simulink model "Quaternions_Method_merge_gio_giusto"  (R2021b)
settings: Solver=FixedStepAuto  StartTime=0.0  StopTime=Time  FixedStep=1  RelTol=1e-13  AbsTol=1e-8
values from neighbouring files (symbols this model uses):
  a = 8.6251e+06    (= 8625100)    [Main.m]
  c = 299792*10^3    (= 299792000)    [Main.m]
  e = 0.1195    [Main.m]
  G = 6.67259 * 1e-11    (= 6.67259e-11)    [Main.m]
  H_0 = sqrt((g_1_0)^2 + (g_1_1)^2 + (h_1_1)^2)    [Main.m]
  i = 0.3815    [Main.m]
  MB = [2000; 0.3; 1; 0.12].*1e-2    [Main.m]
  mr = 1.2 * 0.0001    (= 0.00012)    [Main.m]
  muP = G*Mt    (= 398527110340000)    [Main.m]
  omega_0 = [om_x, om_y, om_z]    [Main.m]
  p_acc = deg2rad(5)    [Main.m]
  RD = 0.1*ones(1,10)    [Main.m]
  RS_MB = 0.5    [Main.m]
  RS_SP = 0.1    [Main.m]
  SP = [2000; 0.3; 1; 0.12].*1e-2    [Main.m]
  theta0 = 0    [Main.m]
  w_E = (2*pi)/(24*3600)    (= 7.27220521664e-05)    [Main.m]
undefined symbols (not defined in the file or in its folder): A_BN_0, A_rw, A_rw_star, H, magnitude, rho_d_MB, rho_d_SP, rho_s_MB, rho_s_SP, sig_b, sig_n, T, t_sample
libraries: matrix_library x23, vrlib x9, simulink_extras x2, simulink x2
(part 1 of 8)
settings Model: SimulationMode=accelerator  Creator=dario  LastModifiedBy=adity
settings SolverCC: ZeroCrossControl=DisableAll  ZeroCrossAlgorithm=Adaptive  AlgebraicLoopSolver=TrustRegion
settings DebuggingCC: IgnoredZcDiagnostic=none

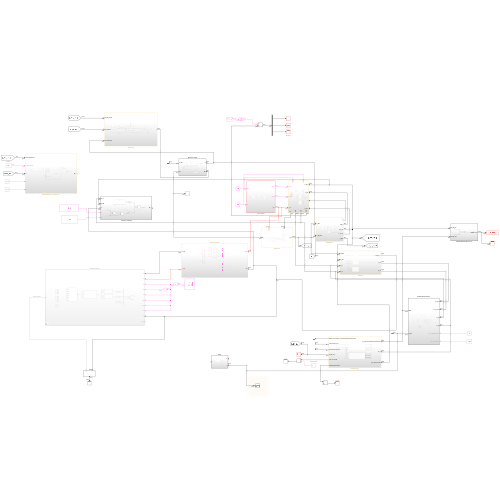
[thumbnail: Simulink's stored preview of the top-level diagram]
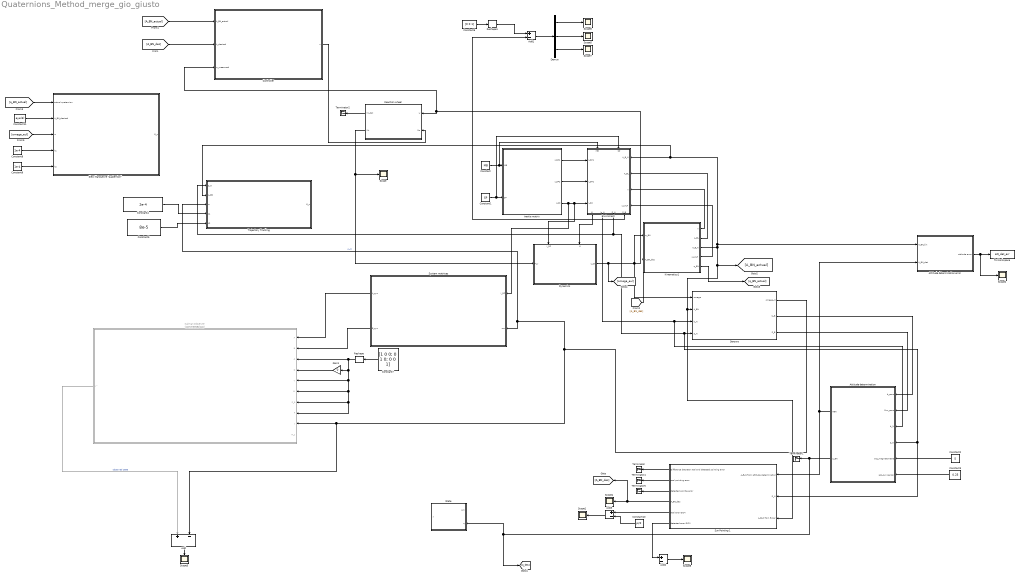
== system Quaternions_Method_merge_gio_giusto ==
  Add{,1..3} (4 alike) : Sum  Inputs=+-
  Attitude determination : Subsystem
  Attitude determination error : Subsystem
  Constant : Constant  Value=MB
  Constant1 : Constant  Value=SP
  Constant10 : Constant  Value=pi/2
  Constant11 : Constant  Value=eye(3)
  Constant2 : Constant  Value=5
  Constant3 : Constant  Value=0.25
  Constant4 : Constant  Value=2e-4
  Constant5 : Constant  Value=8e-5
  Constant6 : Constant  Value=[0 0 1]  VectorParams1D=off
  Constant7 : Constant  Value=[1 0 0; 0 1 0; 0 0 1]  VectorParams1D=off
  Constant8 : Constant  Value=1e-4
  Constant9 : Constant  Value=1e-4
  Controller : Subsystem
  Demux : Demux  Outputs=3
  Dynamics : Subsystem
      settings: PortSchema="{\"entries\":[{\"content\":{\"sides\":[{\"content\":{\"connectorIds\":[\"In1\"]},\"type\":\"ConnectorPlacement.EquallySpacedRectSide\",\"uuid\":\"0fb0fd28-732a-45b7-951f-4b0b2306202c\"},{\"content\":{\"connectorIds\":[\"Out1\"],\"side\":\"RIGHT\"},\"type\":\"ConnectorPlacement.EquallySpacedRectSide\",\"uuid\":\"160a6d95-5e8b-4088-9ac4-372e2ef53b1e\"},{\"content\":{\"connectorIds\":[\"In2\",\"In3\"],\"side\":\"TOP\"},\"type\":\"ConnectorPlacement.EquallySpacedRectSide\",\"uuid\":\"bc0d773d-9b3c-40c2-804a-fc9efd6e220c\"}]},\"type\":\"ConnectorPlacement.EquallySpacedConnector\",\"uuid\":\"1f85a25c-c8d4-4d9d-9994-483d99135538\"}],\"packageUris\":[\"http://schema.mathworks.com/mf0/Connector/R2020b\"],\"version\":\"1.0\"}"
  Enviroment : Subsystem
      settings: PortSchema="{\"entries\":[{\"content\":{\"sides\":[{\"content\":{\"connectorIds\":[\"In1\",\"In2\"]},\"type\":\"ConnectorPlacement.EquallySpacedRectSide\",\"uuid\":\"77a65197-c5ef-4c05-af97-bd670bb59a1b\"},{\"content\":{\"connectorIds\":[\"Out1\",\"Out2\",\"Out3\",\"Out4\"],\"side\":\"RIGHT\"},\"type\":\"ConnectorPlacement.EquallySpacedRectSide\",\"uuid\":\"f4905732-994b-44e8-915f-1f1165b6d340\"},{\"content\":{\"connectorIds\":[\"In3\",\"In4\",\"In5\"],\"side\":\"TOP\"},\"type\":\"ConnectorPlacement.EquallySpacedRectSide\",\"uuid\":\"dbb628bc-072b-4daa-a580-a056bf799753\"},{\"content\":{\"connectorIds\":[\"In6\",\"In7\",\"In8\",\"In9\"],\"side\":\"BOTTOM\"},\"type\":\"ConnectorPlacement.EquallySpacedRectSide\",\"uuid\":\"e6af6235-b92e-4098-9bbc-91b77f168ead\"}]},\"type\":\"ConnectorPlacement.EquallySpacedConnector\",\"uuid\":\"a4645f0d-8f51-4ba7-9ec5-d423e83ccc17\"}],\"packageUris\":[\"http://schema.mathworks.com/mf0/Connector/R2020b\"],\"version\":\"1.0\"}"
  Gain1 : Gain  Gain=0
  Inertia matrix : Subsystem
  Kalman Observer : Subsystem  Commented=on
  Kinematics1 : Subsystem
  Reaction wheel : Subsystem
  Reshape : Reshape  OutputDimensionality=Customize  OutputDimensions=[3,3]
  Reshape1 : Reshape  OutputDimensionality=Column vector (2-D)
  Scope{,1..8} (9 alike) : Scope
  Sensors : Subsystem
  "Slew Manouevre \"quaternion\"" : Subsystem
  State : Subsystem
  Sun Pointing 1 : Subsystem
  System matrices : Subsystem
  Terminator{,1..2,4..5} (5 alike) : Terminator
  To Workspace : ToWorkspace  VariableName=att_det_err  SaveFormat=Timeseries  SampleTime=-1
  Trajectory Tracking : Subsystem
  wires:
  Enviroment/1(M) -> Dynamics/3(M)
  Kinematics1/2(A_BL) -> Enviroment/7(A_BL)
  Kinematics1/1(n) -> Enviroment/8(n)
  Constant/1 -> Inertia matrix/1(MB), Enviroment/1(MB)
  Constant1/1 -> Inertia matrix/2(SP), Enviroment/2(SP)
  Inertia matrix/1(r_SP1) -> Enviroment/3(r_SP1)
  Inertia matrix/2(r_SP2) -> Enviroment/4(r_SP2)
  Dynamics/1(ω_B) -> [omega_eul], Controller/3(w_measured), Reaction wheel/1(w), Kinematics1/1(ω_BN), Sensors/1(omega)
  Inertia matrix/3(I_SC) -> System matrices/1(I_SC), Enviroment/5(I_SC), Dynamics/2(I_SC)
  Sensors/1(omega_m) -> Add/2, Kalman Observer/9(x), Trajectory Tracking/3(" ω"), System matrices/2(om)  "w_m"
  Enviroment/2(b_N) -> Attitude determination/3(b_N), Sensors/3(b_N)
  Enviroment/3(S_N) -> Sun Pointing 1/2(S_N), Attitude determination/4(S_N), Sensors/4(S_N), Trajectory Tracking/1(S_N)
  Constant3/1 -> Attitude determination/6(acc_sun sensor)
  Attitude determination/1(ABN) -> Attitude determination error/2(A_BN_det), Sun Pointing 1/1(A_B_N from attitude determination)
  Sensors/2(b_B) -> Attitude determination/1(b_sens)
  Attitude determination/2(q_BN) -> State/2(q), [q_des], Terminator1/1
  Constant2/1 -> Attitude determination/5(acc_magnetometre)
  Sensors/3(S_B) -> Attitude determination/2(Sun_sens)
  Sun Pointing 1/3(detected pointig error) -> Terminator5/1
  Sun Pointing 1/2(real pointing error) -> Terminator4/1
  Sun Pointing 1/1(Difference between real and detected pointing error) -> Terminator/1
  Kinematics1/4(r_LVLH) -> Enviroment/9(r_LVLH)
  Attitude determination error/1(attitude error) -> Scope2/1, To Workspace/1
  System matrices/1(A_sys) -> Kalman Observer/1(A)
  System matrices/2(B_sys) -> Kalman Observer/2(B)
  Constant7/1 -> Reshape/1
  Gain1/1 -> Kalman Observer/4(D)
  Kalman Observer/1(x^) -> Add/1  "observed state"
  Add/1 -> Scope3/1
  Reshape/1 -> Kalman Observer/3(C), Gain1/1, Kalman Observer/5(V), Kalman Observer/6(W), Kalman Observer/7(P_0), Kalman Observer/8(F)
  Constant4/1 -> Trajectory Tracking/4(k1)
  Constant5/1 -> Trajectory Tracking/5(k2)
  Reaction wheel/2(Mr) -> Dynamics/1(M_r), Scope/1
  Reaction wheel/1(hr_dot) -> Terminator2/1
  Sun Pointing 1/4(A_BN_des) -> [A_BN_des], Scope4/1
  [A_BN_des] -> Controller/2(A_desired)
  [A_BN_actual] -> Controller/1(A_BN_actual)
  Controller/1(u) -> Reaction wheel/2(Mc)
  Kinematics1/3(A_B_N) -> Sun Pointing 1/3(A_B_N from Euler), Sensors/2(A_BN), [A_BN_actual], Trajectory Tracking/2(A_BN), Enviroment/6(A_B_N), Attitude determination error/1(A_BN_kin)
  Constant6/1 -> Reshape1/1
  Enviroment/4(S_B) -> Add1/2
  Reshape1/1 -> Add1/1
  Add1/1 -> Demux/1
  Demux/2 -> Scope5/1
  Demux/1 -> Scope6/1
  Demux/3 -> Scope7/1
  [A_BN_des] -> Kinematics1/2(A_BN_des)
  Sun Pointing 1/6(detected error DCM) -> Add2/1
  Add2/1 -> Scope8/1
  Kinematics1/5(q_BN) -> [q_BN_actual]
  [q_BN_actual] -> "Slew Manouevre \"quaternion\""/1(actual quaternion)
  Constant11/1 -> "Slew Manouevre \"quaternion\""/2(A_BN_desired)
  [omega_eul] -> "Slew Manouevre \"quaternion\""/3(ω)
  Constant9/1 -> "Slew Manouevre \"quaternion\""/5(k2)
  Constant8/1 -> "Slew Manouevre \"quaternion\""/4(k1)
  Sun Pointing 1/5(real error DCM) -> Add3/1
  Add3/1 -> Scope1/1
  Constant10/1 -> Add3/2

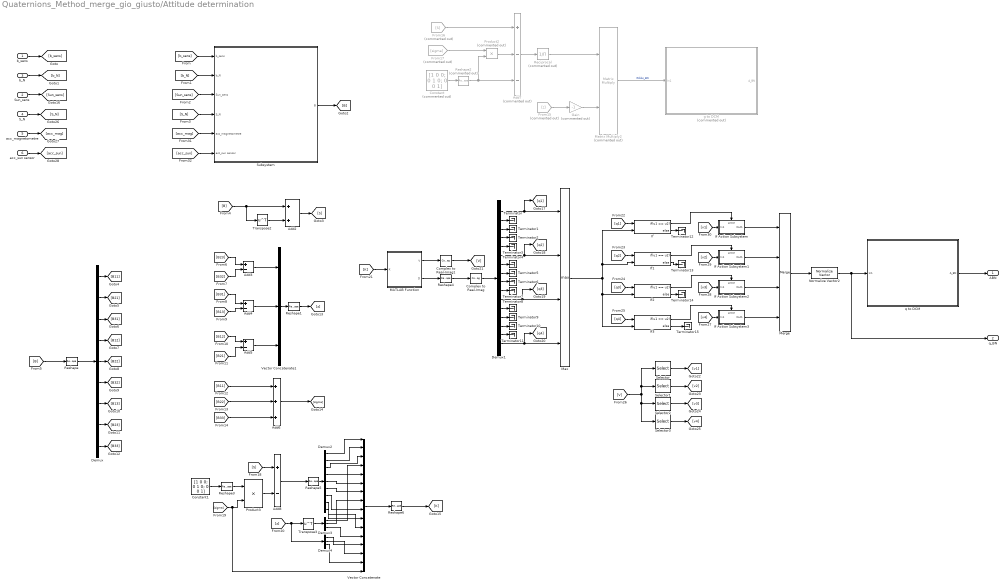
== system Quaternions_Method_merge_gio_giusto/Attitude determination ==
  b_sens : Inport
  Sun_sens : Inport  Port=2
  b_N : Inport  Port=3
  S_N : Inport  Port=4
  acc_magnetometre : Inport  Port=5
  acc_sun sensor : Inport  Port=6
  Add2 : Sum
  Add{3..5,8} (4 alike) : Sum  Inputs=+-
  Add6 : Sum  Inputs=+++
  Add7 : Sum  Commented=on  Inputs=+--
  Complex to Real-Imag : ComplexToRealImag  Output=Real
  Complex to Real-Imag1 : ComplexToRealImag  Output=Real
  Constant : Constant  Commented=on  Value=[1 0 0; 0 1 0; 0 0 1]  VectorParams1D=off
  Constant1 : Constant  Value=[1 0 0; 0 1 0; 0 0 1]  VectorParams1D=off
  Demux : Demux  Outputs=9
  Demux1 : Demux  Outputs=16
  Demux2 : Demux  Outputs=9
  Demux3 : Demux  Outputs=3
  Demux4 : Demux  Outputs=3
  From15 : From  Commented=on  GotoTag=z
  From16 : From  Commented=on  GotoTag=S
  From17 : From  Commented=on  GotoTag=sigma
  Gain : Gain  Commented=on  Gain=-1
  If{,1..3} (4 alike) : If  NumInputs=2  IfExpression=u1 == u2
  If Action Subsystem : Subsystem  TreatAsAtomicUnit=on
  If Action Subsystem1 : Subsystem  TreatAsAtomicUnit=on
  If Action Subsystem2 : Subsystem  TreatAsAtomicUnit=on
  If Action Subsystem3 : Subsystem  TreatAsAtomicUnit=on
  MATLAB Function : MATLAB Function  TreatAsAtomicUnit=on
  Matrix Multiply2 : Product  Commented=on  Multiplication=Matrix(*)
  Max : MinMax  Function=max  Inputs=4
  Merge : Merge  Inputs=4
  Normalize Vector2 : vrlib/Utilities/Normalize Vector  maxzero=0
  Product2 : Product  Commented=on
  Product3 : Product
  Reciprocal : Product  Commented=on  Inputs=/
  Reshape{,1,4..5} (4 alike) : Reshape  OutputDimensionality=Column vector (2-D)
  Reshape2 : Reshape  Commented=on  OutputDimensionality=Customize  OutputDimensions=[3,3]
  Reshape3 : Reshape  OutputDimensionality=Customize  OutputDimensions=[3,3]
  Reshape6 : Reshape  OutputDimensionality=Customize  OutputDimensions=[4,4]
  Selector : Selector  NumberOfDimensions=2  InputPortWidth=3  IndexOptions=Index vector (dialog),Index vector (dialog)  Indices=[1 2 3 4],1  OutputSizes=1,1
  Selector1 : Selector  NumberOfDimensions=2  InputPortWidth=3  IndexOptions=Index vector (dialog),Index vector (dialog)  Indices=[1 2 3 4],2  OutputSizes=1,1
  Selector2 : Selector  NumberOfDimensions=2  InputPortWidth=3  IndexOptions=Index vector (dialog),Index vector (dialog)  Indices=[1 2 3 4],3  OutputSizes=1,1
  Selector3 : Selector  NumberOfDimensions=2  InputPortWidth=3  IndexOptions=Index vector (dialog),Index vector (dialog)  Indices=[1 2 3 4],4  OutputSizes=1,1
  Subsystem : Subsystem
  Terminator{,1..15} (16 alike) : Terminator
  Transpose2 : Math  Operator=transpose  SaturateOnIntegerOverflow=on
  Transpose3 : Math  Operator=transpose  SaturateOnIntegerOverflow=on
  Vector Concatenate : Concatenate  NumInputs=16
  Vector Concatenate1 : Concatenate  NumInputs=3
  g to DCM : Subsystem  Commented=on
  q to DCM : Subsystem
  ABN : Outport
  q_BN : Outport  Port=2
  wires:
  [B] -> Transpose2/1, Add2/1
  Transpose2/1 -> Add2/2
  Add2/1 -> [S]
  [B] -> Reshape/1
  Reshape/1 -> Demux/1
  Demux/1 -> [B11]
  Demux/2 -> [B21]
  Demux/3 -> [B31]
  Demux/4 -> [B12]
  Demux/5 -> [B22]
  Demux/6 -> [B32]
  Demux/7 -> [B13]
  Demux/8 -> [B23]
  Demux/9 -> [B33]
  [B23] -> Add3/1
  [B32] -> Add3/2
  [B31] -> Add4/1
  [B13] -> Add4/2
  [B12] -> Add5/1
  [B21] -> Add5/2
  Add3/1 -> Vector Concatenate1/1
  Add4/1 -> Vector Concatenate1/2
  Add5/1 -> Vector Concatenate1/3
  Vector Concatenate1/1 -> Reshape1/1
  Reshape1/1 -> [z]
  [B11] -> Add6/1
  [B22] -> Add6/2
  [B33] -> Add6/3
  Add6/1 -> [sigma]
  From15/1 -> Gain/1
  Constant/1 -> Reshape2/1
  From17/1 -> Product2/1
  Reshape2/1 -> Add7/3, Product2/2
  From16/1 -> Add7/1
  Product2/1 -> Add7/2
  Add7/1 -> Reciprocal/1
  Reciprocal/1 -> Matrix Multiply2/1
  Gain/1 -> Matrix Multiply2/2
  Matrix Multiply2/1 -> g to DCM/1(In1)  "Gibbs_BN"
  Constant1/1 -> Reshape3/1
  Reshape3/1 -> Product3/1
  [sigma] -> Vector Concatenate/16, Product3/2
  Product3/1 -> Add8/2
  [S] -> Add8/1
  Add8/1 -> Reshape5/1
  MATLAB Function/2(D) -> Reshape4/1
  Demux1/2 -> Terminator/1
  Demux1/3 -> Terminator1/1
  Demux1/4 -> Terminator2/1
  Demux1/5 -> Terminator3/1
  Demux1/6 -> [q2], Max/2
  Demux1/7 -> Terminator4/1
  Demux1/8 -> Terminator5/1
  Demux1/9 -> Terminator6/1
  Demux1/10 -> Terminator7/1
  Demux1/11 -> [q3], Max/3
  Demux1/16 -> [q4], Max/4
  Demux1/12 -> Terminator8/1
  Demux1/13 -> Terminator9/1
  Demux1/14 -> Terminator10/1
  Demux1/15 -> Terminator11/1
  Reshape4/1 -> Complex to Real-Imag/1
  Max/1 -> If3/2, If2/2, If1/2, If/2
  Demux1/1 -> [q1], Max/1
  [q1] -> If/1
  [q2] -> If1/1
  [q4] -> If3/1
  [q3] -> If2/1
  MATLAB Function/1(V) -> Complex to Real-Imag1/1
  Selector1/1 -> [v2]
  Selector3/1 -> [v4]
  Selector2/1 -> [v3]
  Selector/1 -> [v1]
  [V] -> Selector/1, Selector1/1, Selector3/1, Selector2/1
  If/1 -> If Action Subsystem/Action
  If/2 -> Terminator12/1
  If1/2 -> Terminator13/1
  If2/2 -> Terminator14/1
  If3/2 -> Terminator15/1
  If Action Subsystem/1(Out1) -> Merge/1
  If1/1 -> If Action Subsystem1/Action
  If2/1 -> If Action Subsystem2/Action
  If3/1 -> If Action Subsystem3/Action
  If Action Subsystem3/1(Out1) -> Merge/4
  If Action Subsystem2/1(Out1) -> Merge/3
  If Action Subsystem1/1(Out1) -> Merge/2
  [v4] -> If Action Subsystem3/1(In1)
  [v1] -> If Action Subsystem/1(In1)
  [v2] -> If Action Subsystem1/1(In1)
  [v3] -> If Action Subsystem2/1(In1)
  q to DCM/1(A_BN) -> ABN/1
  Merge/1 -> Normalize Vector2/1
  Reshape5/1 -> Demux2/1
  Demux2/1 -> Vector Concatenate/1
  Demux2/2 -> Vector Concatenate/2
  Demux2/3 -> Vector Concatenate/3
  [z] -> Demux4/1, Transpose3/1
  Transpose3/1 -> Demux3/1
  Demux3/1 -> Vector Concatenate/4
  Demux2/4 -> Vector Concatenate/5
  Demux2/5 -> Vector Concatenate/6
  Demux2/6 -> Vector Concatenate/7
  Demux3/2 -> Vector Concatenate/8
  Demux2/7 -> Vector Concatenate/9
  Demux2/8 -> Vector Concatenate/10
  Demux2/9 -> Vector Concatenate/11
  Demux3/3 -> Vector Concatenate/12
  Demux4/2 -> Vector Concatenate/14
  Demux4/1 -> Vector Concatenate/13
  Demux4/3 -> Vector Concatenate/15
  Vector Concatenate/1 -> Reshape6/1
  Reshape6/1 -> [K]
  Complex to Real-Imag/1 -> Demux1/1
  Normalize Vector2/1 -> q_BN/1, q to DCM/1(In1)
  Complex to Real-Imag1/1 -> [V]
  [K] -> MATLAB Function/1(K)
  Subsystem/1(B) -> [B]
  b_sens/1 -> [b_sens]
  b_N/1 -> [b_N]
  Sun_sens/1 -> [Sun_sens]
  S_N/1 -> [S_N]
  acc_magnetometre/1 -> [acc_mag]
  acc_sun sensor/1 -> [acc_sun]
  [b_sens] -> Subsystem/1(b_sens)
  [b_N] -> Subsystem/2(b_N)
  [Sun_sens] -> Subsystem/3(Sun_sens)
  [S_N] -> Subsystem/4(S_N)
  [acc_mag] -> Subsystem/5(acc_magnetometre)
  [acc_sun] -> Subsystem/6(acc_sun sensor)

== system Quaternions_Method_merge_gio_giusto/Attitude determination error ==
  A_BN_kin : Inport
  A_BN_det : Inport  Port=2
  Add : Sum  Inputs=+-
  attitude error : Outport
  wires:
  Add/1 -> attitude error/1
  A_BN_kin/1 -> Add/2
  A_BN_det/1 -> Add/1

== system Quaternions_Method_merge_gio_giusto/Controller ==
  A_BN_actual : Inport
  A_desired : Inport  Port=2
  w_measured : Inport  Port=3
  -k1 : Gain  Gain=-3*10^-5
  -k2 : Gain  Gain=-3*10^-5
  Gain : Gain  Gain=-1
  Matrix Multiply : Product  Multiplication=Matrix(*)
  Mux : Mux  Inputs=3
  Reshape : Reshape  OutputDimensionality=Customize  OutputDimensions=[3,1]
  Scope{,1..3} (4 alike) : Scope
  Selector : Selector  NumberOfDimensions=2  InputPortWidth=3  IndexOptions=Index vector (dialog),Index vector (dialog)  Indices=2,1  OutputSizes=1,1
  Selector1 : Selector  NumberOfDimensions=2  InputPortWidth=3  IndexOptions=Index vector (dialog),Index vector (dialog)  Indices=3,1  OutputSizes=1,1
  Selector2 : Selector  NumberOfDimensions=2  InputPortWidth=3  IndexOptions=Index vector (dialog),Index vector (dialog)  Indices=3,2  OutputSizes=1,1
  Sum : Sum  Inputs=|+|-|
  Sum1 : Sum  Inputs=|+|+|
  Transpose1 : Math  Operator=transpose  SaturateOnIntegerOverflow=on
  u : Outport
  wires:
  A_desired/1 -> Matrix Multiply/2
  A_BN_actual/1 -> Matrix Multiply/1
  Matrix Multiply/1 -> Scope/1, Sum/2, Transpose1/1
  Transpose1/1 -> Sum/1
  Sum/1 -> Selector2/1, Selector/1, Selector1/1
  Mux/1 -> Reshape/1
  Selector1/1 -> Gain/1
  Selector/1 -> Scope3/1, Mux/1
  Selector2/1 -> Mux/3
  -k2/1 -> Sum1/1
  Sum1/1 -> Scope2/1, u/1
  w_measured/1 -> Scope1/1, -k1/1
  -k1/1 -> Sum1/2
  Reshape/1 -> -k2/1
  Gain/1 -> Mux/2

== system Quaternions_Method_merge_gio_giusto/Dynamics ==
  M_r : Inport
  I_SC : Inport  Port=2
  M : Inport  Port=3
  Add : Sum
  Constant7 : Constant  Value=omega_0
  Cross Product : vrlib/Utilities/Cross Product
  Demux : Demux  Outputs=3
  Gain5 : Gain  Gain=-1
  Integrator4 : Integrator  InitialConditionSource=external  InitialCondition=omega_0
  Product6 : Product  Multiplication=Matrix(*)
  Product7 : Product  Multiplication=Matrix(*)
  Reciprocal : Product  Inputs=/  Multiplication=Matrix(*)
  Scope : Scope  NumInputPorts=3
  Sum2 : Sum
  Terminator : Terminator
  ω_B : Outport
  wires:
  Sum2/1 -> Product7/2
  Product6/1 -> Cross Product/2
  Product7/1 -> Terminator/1, Integrator4/1
  Cross Product/1 -> Gain5/1
  Gain5/1 -> Sum2/1
  Integrator4/1 -> Demux/1, Cross Product/1, Product6/2, ω_B/1
  I_SC/1 -> [I_SC]
  [I_SC] -> Product6/1
  [I_SC] -> Reciprocal/1
  Reciprocal/1 -> Product7/1
  Constant7/1 -> [w_0]
  [w_0] -> Integrator4/2
  M/1 -> Add/1
  Demux/2 -> Scope/2  "om_y"
  Demux/1 -> Scope/1  "om_x"
  Demux/3 -> Scope/3  "om_z"
  Add/1 -> Sum2/2
  M_r/1 -> Add/2

== system Quaternions_Method_merge_gio_giusto/Enviroment ==
  MB : Inport
  SP : Inport  Port=2
  r_SP1 : Inport  Port=3
  r_SP2 : Inport  Port=4
  I_SC : Inport  Port=5
  A_B_N : Inport  Port=6
  A_BL : Inport  Port=7
  n : Inport  Port=8
  r_LVLH : Inport  Port=9
  Constant : Constant  Value=6371.2*1e3
  Gravity gradient torque : Subsystem
  "Magnetic torque " : Subsystem
  Scope : Scope
  Scope1 : Scope
  Scope2 : Scope
  Solar Radiation Perturbation : Subsystem  Commented=on
  Solar Radiation Perturbation1 : Subsystem
  Sum : Sum  Inputs=+|+|+
  M : Outport
  b_N : Outport  Port=2
  S_N : Outport  Port=3
  S_B : Outport  Port=4
  wires:
  A_B_N/1 -> Solar Radiation Perturbation1/1(A_B_N), "Magnetic torque "/2(A_B_N)
  MB/1 -> Solar Radiation Perturbation1/2(MB)
  SP/1 -> Solar Radiation Perturbation1/3(SP)
  r_SP1/1 -> Solar Radiation Perturbation1/4(r_SP1)
  r_SP2/1 -> Solar Radiation Perturbation1/5(r_SP2)
  Sum/1 -> M/1
  Solar Radiation Perturbation1/1(M_SRP) -> Scope/1, Sum/2
  "Magnetic torque "/1(M) -> Scope2/1, Sum/3
  Constant/1 -> "Magnetic torque "/1(R)
  Gravity gradient torque/1(M_GG) -> Scope1/1, Sum/1
  I_SC/1 -> Gravity gradient torque/1(I)
  n/1 -> Gravity gradient torque/3(n)
  A_BL/1 -> Gravity gradient torque/2(A_BL)
  "Magnetic torque "/2(b_N) -> [b_N]
  [b_N] -> b_N/1
  Solar Radiation Perturbation1/2(S_N) -> [S_N]
  [S_N] -> S_N/1
  r_LVLH/1 -> "Magnetic torque "/3(r_LVLH)
  Solar Radiation Perturbation1/3(S_B) -> S_B/1

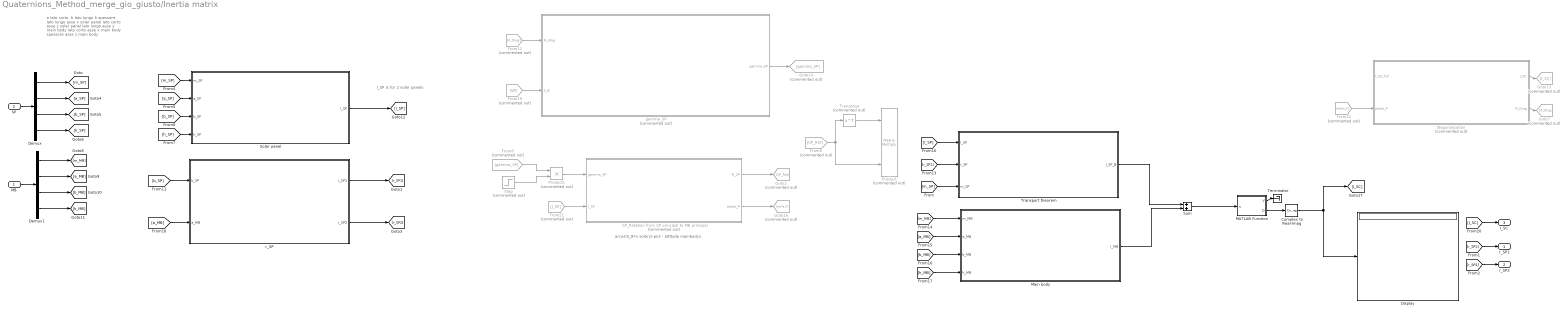
== system Quaternions_Method_merge_gio_giusto/Inertia matrix ==
  note: I_SP is for 2 solar panels
  note: arcos(S_B*n solary)-pi/2 - attitude mainbodyx
  note: a lato corto, b lato lungo h spessore
      | lato lungo asse x solar panel
      | lato corto asse z solar panel
      | lato lungo asse y main body
      | lato corto asse x main body
      | spessore asse z main body
  MB : Inport
  SP : Inport  Port=2
  Complex to Real-Imag : ComplexToRealImag  Output=Real
  Demux : Demux
  Demux1 : Demux
  Diagonalization : Subsystem  Commented=on
  Display : Display
  From12 : From  Commented=on  GotoTag=R_Diag
  From19 : From  Commented=on  GotoTag=SB
  From21 : From  Commented=on  GotoTag=I_SP
  From22 : From  Commented=on  GotoTag=alpha_P
  From8 : From  Commented=on  GotoTag=gamma_SP
  From9 : From  Commented=on  GotoTag=SP_Rot
  Goto13 : Goto  Commented=on  GotoTag=I_SC
  Goto14 : Goto  Commented=on  GotoTag=gamma_SP
  Goto16 : Goto  Commented=on  GotoTag=alpha_P
  Goto2 : Goto  Commented=on  GotoTag=SP_Rot
  Goto7 : Goto  Commented=on  GotoTag=R_Diag
  MATLAB Function : MATLAB Function  TreatAsAtomicUnit=on
  Main body : Subsystem
  Product : Product  Commented=on  Inputs=3  Multiplication=Matrix(*)
  Product1 : Product  Commented=on
  SP_Rotation from SP principal to MB principal : Subsystem  Commented=on
  Solar panel : Subsystem
  Step : Step  Commented=on  Time=1e-3  SampleTime=0
  Sum : Sum
  Terminator : Terminator
  Transport theorem : Subsystem
  Transpose : Math  Commented=on  Operator=transpose  SaturateOnIntegerOverflow=on
  gamma_SP : Subsystem  Commented=on
  r_SP : Subsystem
  r_SP1 : Outport
  r_SP2 : Outport  Port=2
  I_SC : Outport  Port=3
  wires:
  MB/1 -> Demux1/1
  Demux/1 -> [m_SP]
  SP_Rotation from SP principal to MB principal/1(R_SP) -> Goto2/1
  Transpose/1 -> Product/1
  Transport theorem/1(I_SP_B) -> Sum/1
  [r_SP1] -> Transport theorem/2(r_SP)
  Main body/1(I_MB) -> Sum/2
  [m_SP] -> Transport theorem/3(m_SP)
  r_SP/1(r_SP1) -> [r_SP1]
  [r_SP1] -> r_SP1/1
  [r_SP2] -> r_SP2/1
  r_SP/2(r_SP2) -> [r_SP2]
  Demux/2 -> [a_SP]
  Demux/3 -> [b_SP]
  Demux/4 -> [h_SP]
  [a_SP] -> Solar panel/2(a_SP)
  [b_SP] -> Solar panel/3(b_SP)
  [m_SP] -> Solar panel/1(m_SP)
  [h_SP] -> Solar panel/4(h_SP)
  From9/1 -> Transpose/1, Product/3
  [b_SP] -> r_SP/1(b_SP)
  Demux1/4 -> [h_MB]
  Demux1/3 -> [b_MB]
  Demux1/2 -> [a_MB]
  Demux1/1 -> [m_MB]
  [m_MB] -> Main body/1(m_MB)
  [a_MB] -> Main body/2(a_MB)
  [b_MB] -> Main body/3(b_MB)
  [h_MB] -> Main body/4(h_MB)
  [a_MB] -> r_SP/2(a_MB)
  Solar panel/1(I_SP) -> [I_SP]
  Product1/1 -> SP_Rotation from SP principal to MB principal/1(gamma_SP)
  From8/1 -> Product1/1
  Step/1 -> Product1/2
  SP/1 -> Demux/1
  Diagonalization/2(R_Diag) -> Goto7/1
  From12/1 -> gamma_SP/1(R_diag)
  From19/1 -> gamma_SP/2(S_B)
  Diagonalization/1(I_SC) -> Goto13/1
  [I_SC] -> I_SC/1
  gamma_SP/1(gamma_SP) -> Goto14/1
  From21/1 -> SP_Rotation from SP principal to MB principal/2(I_SP)
  SP_Rotation from SP principal to MB principal/2(alpha_P) -> Goto16/1
  From22/1 -> Diagonalization/2(alpha_P)
  [I_SP] -> Transport theorem/1(I_SP)
  Sum/1 -> MATLAB Function/1(u)
  MATLAB Function/1(V) -> Terminator/1
  MATLAB Function/2(D) -> Complex to Real-Imag/1
  Complex to Real-Imag/1 -> [I_SC], Display/1

== system Quaternions_Method_merge_gio_giusto/Kalman Observer ==
  A : Inport
  B : Inport  Port=2
  C : Inport  Port=3
  D : Inport  Port=4
  V : Inport  Port=5
  W : Inport  Port=6
  P_0 : Inport  Port=7
  F : Inport  Port=8
  x : Inport  Port=9
  M_c : Inport  Port=10
  A^ : Subsystem
  Add : Sum  Inputs=+++
  B^ : Subsystem
  Integrator : Integrator  InitialConditionSource=external
  L : Subsystem
  Matrix Multiply : Product  Multiplication=Matrix(*)
  Matrix Multiply1 : Product  Multiplication=Matrix(*)
  Matrix Multiply2 : Product  Multiplication=Matrix(*)
  Riccati : Subsystem
  x^ : Outport
  wires:
  A/1 -> [A]
  V/1 -> [V]
  B/1 -> [B]
  W/1 -> [W]
  F/1 -> [F]
  [A] -> Riccati/1(A)
  [F] -> Riccati/3(F)
  [W] -> Riccati/4(W)
  [V] -> Riccati/5(V)
  [B] -> B^/1(B)
  [L] -> B^/2(L)
  C/1 -> [C]
  [C] -> Riccati/2(C)
  L/1(L) -> [L]
  [P] -> L/1(P)
  Riccati/1(P) -> [P]
  [C] -> L/2(C)
  [V] -> L/3(V)
  [A] -> A^/1(A)
  [L] -> A^/2(L)
  x/1 -> [x]
  A^/1(A^) -> Matrix Multiply/1
  [x_obs] -> Matrix Multiply/2
  B^/1(B^) -> Matrix Multiply1/1
  M_c/1 -> [M_c]
  [M_c] -> Matrix Multiply1/2
  Matrix Multiply1/1 -> Add/1
  Matrix Multiply/1 -> Add/2
  Add/1 -> Integrator/1
  Integrator/1 -> [x_obs], x^/1
  [L] -> Matrix Multiply2/1
  [x] -> Matrix Multiply2/2
  [x] -> Integrator/2
  P_0/1 -> [P_0]
  [P_0] -> Riccati/6(P_0)
  D/1 -> [D]
  [D] -> B^/3(D)
  [C] -> A^/3(C)
  Matrix Multiply2/1 -> Add/3

== system Quaternions_Method_merge_gio_giusto/Kinematics1 ==
  ω_BN : Inport
  A_BN_des : Inport  Port=2
  Creazione Matrice A_BN : Subsystem
  Creazione quaternione : Subsystem
  MatrixMultiply : Product  Multiplication=Matrix(*)
  Orbit Propagation : Subsystem
  Relative_Attitude : Subsystem
  n : Outport
  A_BL : Outport  Port=2
  A_B_N : Outport  Port=3
  r_LVLH : Outport  Port=4
  q_BN : Outport  Port=5
  wires:
  Creazione Matrice A_BN/1(A_BN) -> A_B_N/1, Relative_Attitude/1(A_BN), Orbit Propagation/1(A_BN)
  ω_BN/1 -> Creazione quaternione/1(ω_BN)
  Creazione quaternione/1(q_normalizzato) -> q_BN/1, Creazione Matrice A_BN/1(q_normalizzato)
  Relative_Attitude/1(A_BL) -> A_BL/1
  Orbit Propagation/2(n) -> n/1
  Orbit Propagation/1(theta) -> Relative_Attitude/2(theta)
  Relative_Attitude/2(A_L/N) -> [A_LN]
  Orbit Propagation/3(r_N) -> MatrixMultiply/2
  [A_LN] -> MatrixMultiply/1
  MatrixMultiply/1 -> r_LVLH/1
  A_BN_des/1 -> Creazione quaternione/2(A_BN_des)

== system Quaternions_Method_merge_gio_giusto/Reaction wheel ==
  w : Inport
  Mc : Inport  Port=2
  A : Constant  Value=A_rw
  A_star : Constant  Value=A_rw_star
  Constant : Constant  Value=[0 0 0 0]
  Cross Product : matrix_library/Cross Product
      settings: SourceProductBaseCode=SL
  Gain : Gain  Gain=-1
  Integrator : Integrator  InitialConditionSource=external
  Matrix Multiply : Product  Multiplication=Matrix(*)
  Matrix Multiply1 : Product  Multiplication=Matrix(*)
  Matrix Multiply2 : Product  Multiplication=Matrix(*)
  Reshape : Reshape  OutputDimensionality=Column vector (2-D)
  Reshape1 : Reshape  OutputDimensionality=Column vector (2-D)
  Sum : Sum  Inputs=|++
  hr_dot : Outport
  Mr : Outport  Port=2
  wires:
  Integrator/1 -> Matrix Multiply/2
  A/1 -> [A_rw], Matrix Multiply/1
  w/1 -> Cross Product/1
  Matrix Multiply/1 -> Cross Product/2
  Cross Product/1 -> Sum/1
  Mc/1 -> Reshape1/1
  Sum/1 -> Matrix Multiply1/2
  A_star/1 -> Gain/1
  Gain/1 -> Matrix Multiply1/1
  Matrix Multiply1/1 -> Integrator/1, Matrix Multiply2/2, hr_dot/1
  Constant/1 -> Reshape/1
  Reshape/1 -> Integrator/2
  Reshape1/1 -> Sum/2
  Matrix Multiply2/1 -> Mr/1
  [A_rw] -> Matrix Multiply2/1

== system Quaternions_Method_merge_gio_giusto/Sensors ==
  omega : Inport
  A_BN : Inport  Port=2
  b_N : Inport  Port=3
  S_N : Inport  Port=4
  Gyroscopes : Subsystem
  Magnetometer1 : Subsystem
  Sun sensor : Subsystem
  omega_m : Outport
  b_B : Outport  Port=2
  S_B : Outport  Port=3
  wires:
  omega/1 -> Gyroscopes/1(omega)
  Gyroscopes/1(omega_m) -> omega_m/1
  b_N/1 -> Magnetometer1/2(b_N)
  Magnetometer1/1(b_B) -> b_B/1
  Sun sensor/1(S_B) -> S_B/1
  A_BN/1 -> Sun sensor/2(A_BN), Magnetometer1/1(A_BN)
  S_N/1 -> Sun sensor/1(S_N)

== system Quaternions_Method_merge_gio_giusto/Slew Manouevre "quaternion" ==
  actual quaternion : Inport
  A_BN_desired : Inport  Port=2
  ω : Inport  Port=3
  k1 : Inport  Port=4
  k2 : Inport  Port=5
  A_BN to quaternion : Subsystem
  Creation of Q_euler1 : Subsystem
  Demux : Demux
  Gain : Gain  Gain=-1
  Gain1 : Gain  Gain=-2
  Mux : Mux  Inputs=3
  Product : Product  Multiplication=Matrix(*)
  Product1 : Product
  Product2 : Product  Inputs=3
  Reshape : Reshape  OutputDimensionality=Column vector (2-D)
  Scope : Scope
  Sum : Sum  Inputs=|+|+|
  M_c : Outport
  wires:
  actual quaternion/1 -> Product/2
  Creation of Q_euler1/1(Q_desired) -> Product/1
  A_BN_desired/1 -> A_BN to quaternion/1(" A_BN_Desiderd")
  A_BN to quaternion/1(q_desiderd) -> Creation of Q_euler1/1(q_desired)
  k1/1 -> Gain/1
  Gain/1 -> Product1/1
  ω/1 -> Product1/2
  k2/1 -> Product2/1
  [q_error] -> Product2/3
  Product1/1 -> Sum/1
  Product2/1 -> Sum/2
  Sum/1 -> M_c/1
  Product/1 -> Scope/1, Demux/1
  Demux/1 -> [qe1]
  Demux/4 -> [qe4]
  Demux/3 -> [qe3]
  Demux/2 -> [qe2]
  [qe1] -> Mux/1
  [qe2] -> Mux/2
  [qe3] -> Mux/3
  Mux/1 -> Reshape/1
  Reshape/1 -> [q_error]
  [qe4] -> Gain1/1
  Gain1/1 -> Product2/2

== system Quaternions_Method_merge_gio_giusto/State ==
  om : Inport
  q : Inport  Port=2
  Reshape : Reshape  OutputDimensionality=Column vector (2-D)
  Vector Concatenate : Concatenate
  q to g : Subsystem
  x : Outport
  wires:
  q/1 -> q to g/1(q)
  om/1 -> Vector Concatenate/2
  q to g/1(g) -> Vector Concatenate/1
  Vector Concatenate/1 -> Reshape/1
  Reshape/1 -> x/1

== system Quaternions_Method_merge_gio_giusto/Sun Pointing 1 ==
  A_B_N from attitude determination : Inport
  S_N : Inport  Port=2
  A_B_N from Euler : Inport  Port=3
  Pointing error with DCM : Subsystem
  Pointing error with quaternions : Subsystem
  Difference between real and detected pointing error : Outport
  real pointing error : Outport  Port=2
  detected pointig error : Outport  Port=3
  A_BN_des : Outport  Port=4
  real error DCM : Outport  Port=5
  detected error DCM : Outport  Port=6
  wires:
  A_B_N from attitude determination/1 -> Pointing error with quaternions/1(A_B_N from attitude determination), Pointing error with DCM/3(A_B_N from Euler)
  S_N/1 -> Pointing error with quaternions/2(S_N), Pointing error with DCM/2(S_N)
  A_B_N from Euler/1 -> Pointing error with quaternions/3(A_B_N from Euler), Pointing error with DCM/1(A_B_N from attitude determination)
  Pointing error with DCM/1(Difference between real and detected pointing error) -> Difference between real and detected pointing error/1
  Pointing error with quaternions/2(detected pointing error) -> detected pointig error/1
  Pointing error with quaternions/1(real pointing error) -> real pointing error/1
  Pointing error with quaternions/3(q_euler) -> ?
  Pointing error with quaternions/4(q_desired) -> ?
  Pointing error with quaternions/5(A_BN_des) -> A_BN_des/1
  Pointing error with DCM/2(real error DCM) -> real error DCM/1
  Pointing error with DCM/3(Detected error DCM) -> detected error DCM/1

== system Quaternions_Method_merge_gio_giusto/System matrices ==
  I_SC : Inport
  om : Inport  Port=2
  Add : Sum  Inputs=+-
  Add1 : Sum  Inputs=+-
  Demux : Demux  Outputs=9
  Demux1 : Demux  Outputs=3
  Ground : Ground
  Ground1 : Ground
  Product{,1..3} (4 alike) : Product
  Reciprocal{,1..4} (5 alike) : Product  Inputs=/
  Reshape : Reshape
  Reshape1 : Reshape  OutputDimensionality=Customize  OutputDimensions=[3,3]
  Reshape2 : Reshape  OutputDimensionality=Customize  OutputDimensions=[3,3]
  Terminator{,1..7} (8 alike) : Terminator
  Vector Concatenate : Concatenate  NumInputs=9
  Vector Concatenate1 : Concatenate  NumInputs=9
  A_sys : Outport
  B_sys : Outport  Port=2
  wires:
  I_SC/1 -> Reshape/1
  Reshape/1 -> Demux/1
  Demux/1 -> [I_x]
  Demux/9 -> [I_z]
  Demux/5 -> [I_y]
  Demux/2 -> Terminator/1
  Demux/4 -> Terminator2/1
  Demux/3 -> Terminator1/1
  Demux/6 -> Terminator3/1
  Demux/7 -> Terminator4/1
  Demux/8 -> Terminator5/1
  [I_x] -> Reciprocal/1
  [I_y] -> Reciprocal1/1
  [I_z] -> Reciprocal2/1
  Reciprocal2/1 -> Vector Concatenate1/9
  Reciprocal1/1 -> Vector Concatenate1/5
  Reciprocal/1 -> Vector Concatenate1/1
  Vector Concatenate1/1 -> Reshape1/1
  Reshape1/1 -> B_sys/1
  om/1 -> Demux1/1
  Demux1/2 -> Terminator7/1
  Demux1/3 -> [om_z]
  Reshape2/1 -> A_sys/1
  Vector Concatenate/1 -> Reshape2/1
  Ground/1 -> Vector Concatenate/9, Vector Concatenate/8, Vector Concatenate/7, Vector Concatenate/6, Vector Concatenate/5, Vector Concatenate/3, Vector Concatenate/1
  [I_z] -> Add/1
  [I_x] -> Add/2
  [I_y] -> Reciprocal3/1
  Reciprocal3/1 -> Product/2
  Add/1 -> Product/1
  Add1/1 -> Product1/1
  Reciprocal4/1 -> Product1/2
  [I_z] -> Add1/2
  [I_y] -> Add1/1
  [I_x] -> Reciprocal4/1
  [A_21] -> Vector Concatenate/2
  [A_12] -> Vector Concatenate/4
  Demux1/1 -> Terminator6/1
  Product2/1 -> [A_21]
  Product/1 -> Product2/1
  [om_z] -> Product2/2
  [om_z] -> Product3/2
  Product1/1 -> Product3/1
  Product3/1 -> [A_12]
  Ground1/1 -> Vector Concatenate1/8, Vector Concatenate1/7, Vector Concatenate1/6, Vector Concatenate1/4, Vector Concatenate1/3, Vector Concatenate1/2

== system Quaternions_Method_merge_gio_giusto/Trajectory Tracking ==
  S_N : Inport
  A_BN : Inport  Port=2
  " ω" : Inport  Port=3
  k1 : Inport  Port=4
  k2 : Inport  Port=5
  Cross Product : matrix_library/Cross Product
      settings: SourceProductBaseCode=SL
  Gain : Gain  Gain=-1
  Gain1 : Gain  Gain=-1
  Matrix Multiply : Product  Multiplication=Matrix(*)
  Product : Product
  Product1 : Product
  Sum : Sum  Inputs=|+|+|
  M_c : Outport
  wires:
  S_N/1 -> Cross Product/2, Matrix Multiply/2
  A_BN/1 -> Matrix Multiply/1
  k1/1 -> Gain/1
  k2/1 -> Gain1/1
  Matrix Multiply/1 -> Cross Product/1
  Cross Product/1 -> Product/2
  Gain1/1 -> Product/1
  Gain/1 -> Product1/1
  " ω"/1 -> Product1/2
  Product1/1 -> Sum/1
  Product/1 -> Sum/2
  Sum/1 -> M_c/1

== system Quaternions_Method_merge_gio_giusto/Attitude determination/If Action Subsystem ==
  In1 : Inport
  Action Port : ActionPort  ActionPortLabel=if(u1 == u2)
  Out1 : Outport
  wires:
  In1/1 -> Out1/1

== system Quaternions_Method_merge_gio_giusto/Attitude determination/If Action Subsystem1 ==
  In1 : Inport
  Action Port : ActionPort  ActionPortLabel=if(u1 == u2)
  Out1 : Outport
  wires:
  In1/1 -> Out1/1

== system Quaternions_Method_merge_gio_giusto/Attitude determination/If Action Subsystem2 ==
  In1 : Inport
  Action Port : ActionPort  ActionPortLabel=if(u1 == u2)
  Out1 : Outport
  wires:
  In1/1 -> Out1/1

== system Quaternions_Method_merge_gio_giusto/Attitude determination/If Action Subsystem3 ==
  In1 : Inport
  Action Port : ActionPort  ActionPortLabel=if(u1 == u2)
  Out1 : Outport
  wires:
  In1/1 -> Out1/1

== system Quaternions_Method_merge_gio_giusto/Attitude determination/Subsystem ==
  b_sens : Inport
  b_N : Inport  Port=2
  Sun_sens : Inport  Port=3
  S_N : Inport  Port=4
  acc_magnetometre : Inport  Port=5
  acc_sun sensor : Inport  Port=6
  Add : Sum
  Add1 : Sum
  Divide : Product  Inputs=*/
  Divide1 : Product  Inputs=*/
  Matrix Multiply : Product  Multiplication=Matrix(*)
  Matrix Multiply1 : Product  Multiplication=Matrix(*)
  Normalize Vector : vrlib/Utilities/Normalize Vector  maxzero=0
  Normalize Vector1 : vrlib/Utilities/Normalize Vector  maxzero=0
  Product : Product
  Product1 : Product
  Transpose : Math  Operator=transpose  SaturateOnIntegerOverflow=on
  Transpose1 : Math  Operator=transpose  SaturateOnIntegerOverflow=on
  B : Outport
  wires:
  Transpose/1 -> Matrix Multiply1/2
  b_N/1 -> Normalize Vector1/1
  S_N/1 -> Transpose1/1
  Divide1/1 -> Product1/2
  Normalize Vector/1 -> Matrix Multiply1/1
  Add/1 -> B/1
  Divide/1 -> Product/2
  Product/1 -> Add/1
  b_sens/1 -> Normalize Vector/1
  Add1/1 -> Divide/2, Divide1/2
  [alpha2] -> Divide1/1
  [alpha1] -> Divide/1
  [alpha1] -> Add1/1
  Transpose1/1 -> Matrix Multiply/2
  acc_sun sensor/1 -> [alpha2]
  Matrix Multiply/1 -> Product1/1
  Matrix Multiply1/1 -> Product/1
  [alpha2] -> Add1/2
  acc_magnetometre/1 -> [alpha1]
  Normalize Vector1/1 -> Transpose/1
  Product1/1 -> Add/2
  Sun_sens/1 -> Matrix Multiply/1

== system Quaternions_Method_merge_gio_giusto/Attitude determination/g to DCM ==
  In1 : Inport
  A_BN : Outport
  wires:
  In1/1 -> A_BN/1

== system Quaternions_Method_merge_gio_giusto/Attitude determination/q to DCM ==
  In1 : Inport
  Add : Sum  Inputs=+-
  Add1 : Sum  Inputs=++-
  Constant : Constant  Value=[1 0 0; 0 1 0; 0 0 1]  VectorParams1D=off
  Demux : Demux
  Gain : Gain  Gain=2
  Gain1 : Gain  Gain=2
  Matrix Multiply : Product  Multiplication=Matrix(*)
  Matrix Multiply2 : Product  Multiplication=Matrix(*)
  Mux : Mux  Inputs=3
  Product : Product
  Product1 : Product
  Reshape : Reshape  OutputDimensionality=Column vector (2-D)
  Reshape1 : Reshape  OutputDimensionality=Customize  OutputDimensions=[3,3]
  Square : Math  Operator=square  SaturateOnIntegerOverflow=on
  Transpose : Math  Operator=transpose  SaturateOnIntegerOverflow=on
  Transpose1 : Math  Operator=transpose  SaturateOnIntegerOverflow=on
  q_cross : Subsystem
  A_BN : Outport
  wires:
  In1/1 -> Demux/1
  Demux/4 -> [q4]
  Demux/1 -> [q1]
  Demux/2 -> [q2]
  Demux/3 -> [q3]
  [q4] -> Square/1
  [q2] -> Mux/2
  [q3] -> Mux/3
  [q1] -> Mux/1
  Mux/1 -> Reshape/1
  Reshape/1 -> [q_vect]
  [q_vect] -> Matrix Multiply/2, Transpose/1
  Transpose/1 -> Matrix Multiply/1
  Matrix Multiply/1 -> Add/2
  Square/1 -> Add/1
  Constant/1 -> Reshape1/1
  Reshape1/1 -> Product1/2
  Product1/1 -> Add1/1
  Matrix Multiply2/1 -> Gain/1
  Gain/1 -> Add1/2
  Transpose1/1 -> Matrix Multiply2/2
  [q_vect] -> Transpose1/1, Matrix Multiply2/1
  Gain1/1 -> Add1/3
  Product/1 -> Gain1/1
  [q4] -> Product/2
  q_cross/1(q_cross) -> Product/1
  Add1/1 -> A_BN/1
  [q_vect] -> q_cross/1(q_vect)
  Add/1 -> Product1/1

== system Quaternions_Method_merge_gio_giusto/Enviroment/Gravity gradient torque ==
  I : Inport
  A_BL : Inport  Port=2
  n : Inport  Port=3
  Constant : Constant  Value=3
  Constant1 : Constant  Value=[1 0 0]
  Demux : Demux  Outputs=9
  Demux1 : Demux  Outputs=3
  Matrix Multiply : Product  Multiplication=Matrix(*)
  Mux : Mux  Inputs=3
  Product{,1..9} (10 alike) : Product
  Reshape : Reshape  OutputDimensionality=Column vector (2-D)
  Reshape1 : Reshape  OutputDimensionality=Column vector (2-D)
  Reshape2 : Reshape  OutputDimensionality=Column vector (2-D)
  Square : Math  Operator=square  SaturateOnIntegerOverflow=on
  Sum : Sum  Inputs=+-
  Sum1 : Sum  Inputs=+-
  Sum2 : Sum  Inputs=+-
  Terminator{,1..5} (6 alike) : Terminator
  M_GG : Outport
  wires:
  Demux/4 -> Terminator2/1
  n/1 -> Square/1
  Demux1/1 -> Product5/2, Product7/2
  Demux/2 -> Terminator/1
  Product6/1 -> Product9/1
  Sum/1 -> Product1/1
  Product1/1 -> Product6/1
  Demux/7 -> Terminator4/1
  Demux1/3 -> Product6/2, Product8/2
  Demux/1 -> Sum1/1
  Product5/1 -> Product8/1
  Demux/3 -> Terminator1/1
  I/1 -> Reshape1/1
  Matrix Multiply/1 -> Demux1/1
  Demux/9 -> Sum2/2, Sum1/2, Sum/1
  Constant1/1 -> Reshape/1
  Sum1/1 -> Product2/1
  Sum2/1 -> Product3/1
  Product7/1 -> Mux/3
  Mux/1 -> Reshape2/1
  Demux/5 -> Sum/2, Sum2/1
  Demux/8 -> Terminator5/1
  A_BL/1 -> Matrix Multiply/1
  Product4/1 -> Product7/1
  Product8/1 -> Mux/2
  Demux/6 -> Terminator3/1
  Demux1/2 -> Product4/2, Product9/2
  Product2/1 -> Product5/1
  Product9/1 -> Mux/1
  Product3/1 -> Product4/1
  Reshape/1 -> Matrix Multiply/2
  Reshape1/1 -> Demux/1
  Reshape2/1 -> M_GG/1
  Square/1 -> Product/1
  Product/1 -> Product2/2, Product1/2, Product3/2
  Constant/1 -> Product/2

== system Quaternions_Method_merge_gio_giusto/Enviroment/Magnetic torque  ==
  R : Inport
  A_B_N : Inport  Port=2
  r_LVLH : Inport  Port=3
  Creation of parasitic torque : Subsystem
  Cross Product : matrix_library/Cross Product
      settings: SourceProductBaseCode=SL
  Magnetic field in body frame : Subsystem
  M : Outport
  b_N : Outport  Port=2
  wires:
  R/1 -> Magnetic field in body frame/2(R)
  A_B_N/1 -> Magnetic field in body frame/1(A_B_N)
  Magnetic field in body frame/1(b_B) -> Cross Product/2
  Cross Product/1 -> M/1
  Creation of parasitic torque/1(m) -> Cross Product/1
  Magnetic field in body frame/2(b_N) -> b_N/1
  r_LVLH/1 -> Magnetic field in body frame/3(r_LVLH)

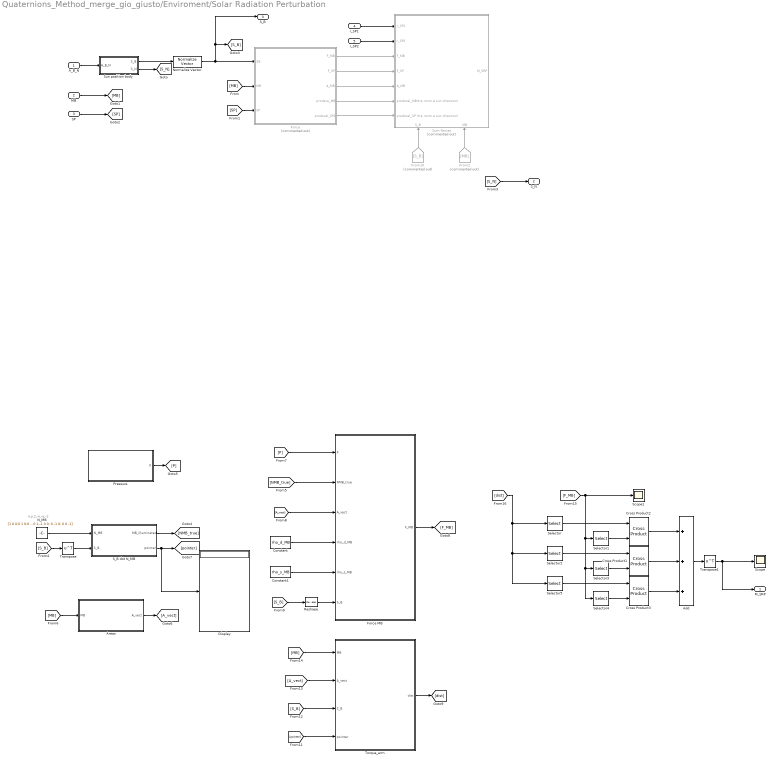
== system Quaternions_Method_merge_gio_giusto/Enviroment/Solar Radiation Perturbation ==
  note: x,y,z,-x,-y,-z
  A_B_N : Inport
  MB : Inport  Port=2
  SP : Inport  Port=3
  r_SP1 : Inport  Port=4
  r_SP2 : Inport  Port=5
  Add : Sum  Inputs=3
  Areas : Subsystem
  Constant : Constant  Value=rho_d_MB
  Constant1 : Constant  Value=rho_s_MB
  Cross Product1 : matrix_library/Cross Product
      settings: SourceProductBaseCode=SL
  Cross Product2 : matrix_library/Cross Product
      settings: SourceProductBaseCode=SL
  Cross Product3 : matrix_library/Cross Product
      settings: SourceProductBaseCode=SL
  Display : Display
  Force : Subsystem  Commented=on
  Force MB : Subsystem
  From10 : From  Commented=on  GotoTag=S_B
  From2 : From  Commented=on  GotoTag=MB
  N_MB : Constant  Value=[1 0 0;0 1 0;0 0 1;-1 0 0; 0 -1 0; 0 0 -1]
  Normalize Vector : vrlib/Utilities/Normalize Vector  maxzero=0
  Pressure : Subsystem
  Reshape : Reshape  OutputDimensionality=Column vector (2-D)
  S_B dot N_MB : Subsystem
  Scope : Scope
  Scope1 : Scope
  Selector : Selector  NumberOfDimensions=2  InputPortWidth=3  IndexOptions=Index vector (dialog),Index vector (dialog)  Indices=1,[1 2 3]  OutputSizes=1,1
  Selector1 : Selector  NumberOfDimensions=2  InputPortWidth=3  IndexOptions=Index vector (dialog),Index vector (dialog)  Indices=1,[1 2 3]  OutputSizes=1,1
  Selector2 : Selector  NumberOfDimensions=2  InputPortWidth=3  IndexOptions=Index vector (dialog),Index vector (dialog)  Indices=2,[1 2 3]  OutputSizes=1,1
  Selector3 : Selector  NumberOfDimensions=2  InputPortWidth=3  IndexOptions=Index vector (dialog),Index vector (dialog)  Indices=2,[1 2 3]  OutputSizes=1,1
  Selector4 : Selector  NumberOfDimensions=2  InputPortWidth=3  IndexOptions=Index vector (dialog),Index vector (dialog)  Indices=3,[1 2 3]  OutputSizes=1,1
  Selector5 : Selector  NumberOfDimensions=2  InputPortWidth=3  IndexOptions=Index vector (dialog),Index vector (dialog)  Indices=3,[1 2 3]  OutputSizes=1,1
  Sum forces : Subsystem  Commented=on
      settings: PortSchema="{\"entries\":[{\"content\":{\"sides\":[{\"content\":{\"connectorIds\":[\"In1\",\"In2\",\"In3\",\"In4\",\"In5\",\"In6\",\"In7\"]},\"type\":\"ConnectorPlacement.EquallySpacedRectSide\",\"uuid\":\"5acb7d4f-0337-4224-9758-4598a3a00165\"},{\"content\":{\"connectorIds\":[\"Out1\"],\"side\":\"RIGHT\"},\"type\":\"ConnectorPlacement.EquallySpacedRectSide\",\"uuid\":\"e6f98c05-9b5f-4378-b9e9-dabff353d596\"},{\"content\":{\"connectorIds\":[],\"side\":\"TOP\"},\"type\":\"ConnectorPlacement.EquallySpacedRectSide\",\"uuid\":\"88e90ea7-7ab4-48d4-8e3b-8712b3a0b993\"},{\"content\":{\"connectorIds\":[\"In8\",\"In9\"],\"side\":\"BOTTOM\"},\"type\":\"ConnectorPlacement.EquallySpacedRectSide\",\"uuid\":\"ececea6a-2c27-462e-a638-503b4beb3cbf\"}]},\"type\":\"ConnectorPlacement.EquallySpacedConnector\",\"uuid\":\"86da1db6-5ce7-4d9e-9b5c-c43957a7360d\"}],\"packageUris\":[\"http://schema.mathworks.com/mf0/Connector/R2020b\"],\"version\":\"1.0\"}"
  Sun position body : Subsystem
  Torque_arm : Subsystem
  Transpose : Math  Operator=transpose  SaturateOnIntegerOverflow=on
  Transpose1 : Math  Operator=transpose  SaturateOnIntegerOverflow=on
  M_SRP : Outport
  S_N : Outport  Port=2
  S_B : Outport  Port=3
  wires:
  A_B_N/1 -> Sun position body/1(A_B_N)
  Sun position body/1(S_B) -> Normalize Vector/1
  Normalize Vector/1 -> S_B/1, [S_B], Force/1(SB)
  Force/3(A_MB) -> Sum forces/5(A_MB)
  Force/1(F_MB) -> Sum forces/3(F_MB)
  r_SP1/1 -> Sum forces/1(r_SP1)
  r_SP2/1 -> Sum forces/2(r_SP2)
  Force/5(prodscal_SP1) -> Sum forces/7(prodscal_SP (tra norm e sun direction))
  Force/4(prodsca_MB) -> Sum forces/6(prodscal_MB(tra norm e sun direction))
  MB/1 -> [MB]
  SP/1 -> [SP]
  [MB] -> Force/2(MB)
  [SP] -> Force/3(SP)
  From2/1 -> Sum forces/9(MB)
  Force/2(F_SP) -> Sum forces/4(F_SP)
  Sun position body/2(S_N) -> [S_N]
  [S_N] -> S_N/1
  N_MB/1 -> S_B dot N_MB/1(N_MB)
  S_B dot N_MB/1(MB_illuminated) -> [NMB_true]
  [NMB_true] -> Force MB/2(NMB_true)
  [S_B] -> Transpose/1
  Transpose/1 -> S_B dot N_MB/2(S_B)
  [MB] -> Areas/1(MB)
  Pressure/1(P) -> [P]
  Areas/1(A_vect) -> [A_vect]
  [P] -> Force MB/1(P)
  [A_vect] -> Force MB/3(A_vect)
  Constant/1 -> Force MB/4(rho_d_MB)
  Constant1/1 -> Force MB/5(rho_s_MB)
  [S_B] -> Reshape/1
  From10/1 -> Sum forces/8(S_B)
  S_B dot N_MB/2(pointer) -> Display/1, [pointer]
  [pointer] -> Torque_arm/4(pointer)
  [S_B] -> Torque_arm/3(S_B)
  [A_vect] -> Torque_arm/2(A_vect)
  [MB] -> Torque_arm/1(MB)
  Reshape/1 -> Force MB/6(S_B)
  Cross Product2/1 -> Add/1
  Selector/1 -> Cross Product2/1
  Selector1/1 -> Cross Product2/2
  Selector3/1 -> Cross Product1/2
  Selector2/1 -> Cross Product1/1
  [dist] -> Selector2/1, Selector5/1, Selector/1
  Cross Product1/1 -> Add/2
  Force MB/1(F_MB) -> [F_MB]
  [F_MB] -> Scope1/1, Selector4/1, Selector3/1, Selector1/1
  Cross Product3/1 -> Add/3
  Selector4/1 -> Cross Product3/2
  Selector5/1 -> Cross Product3/1
  Add/1 -> Transpose1/1
  Torque_arm/1(dist) -> [dist]
  Transpose1/1 -> M_SRP/1, Scope/1

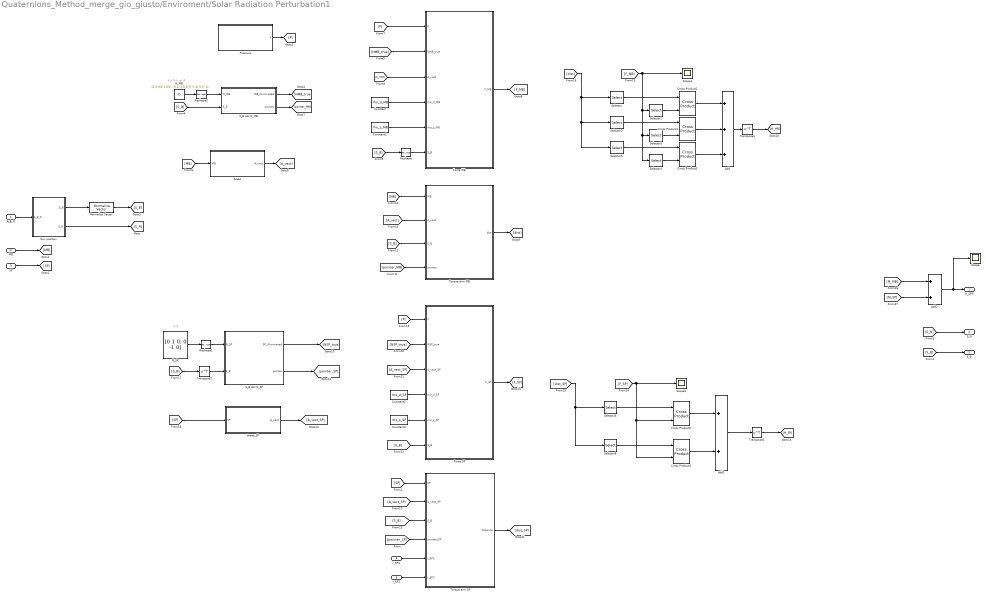
== system Quaternions_Method_merge_gio_giusto/Enviroment/Solar Radiation Perturbation1 ==
  note: x,y,z,-x,-y,-z
  note: y,-y
  A_B_N : Inport
  MB : Inport  Port=2
  SP : Inport  Port=3
  r_SP1 : Inport  Port=4
  r_SP2 : Inport  Port=5
  Add : Sum  Inputs=3
  Add1 : Sum
  Add2 : Sum
  Areas : Subsystem
  Areas_SP : Subsystem
  Constant : Constant  Value=rho_d_MB
  Constant1 : Constant  Value=rho_s_MB
  Constant2 : Constant  Value=rho_d_SP
  Constant3 : Constant  Value=rho_s_SP
  Cross Product{1..5} (5 alike) : matrix_library/Cross Product
      settings: SourceProductBaseCode=SL
  Force MB : Subsystem
  Force SP : Subsystem
  N_MB : Constant  Value=[1 0 0;0 1 0;0 0 1;-1 0 0; 0 -1 0; 0 0 -1]  VectorParams1D=off
  N_SP : Constant  Value=[0 1 0; 0 -1 0]  VectorParams1D=off
  Normalize Vector : vrlib/Utilities/Normalize Vector  maxzero=0
  Pressure : Subsystem
  Reshape : Reshape  OutputDimensionality=Column vector (2-D)
  Reshape1 : Reshape  OutputDimensionality=Customize  OutputDimensions=[2,3]
  Reshape2 : Reshape  OutputDimensionality=Customize  OutputDimensions=[6,3]
  S_B dot N_MB : Subsystem
  S_B dot N_SP : Subsystem
  Scope : Scope
  Scope1 : Scope
  Scope3 : Scope
  Selector : Selector  NumberOfDimensions=2  InputPortWidth=3  IndexOptions=Index vector (dialog),Index vector (dialog)  Indices=1,[1 2 3]  OutputSizes=1,1
  Selector1 : Selector  NumberOfDimensions=2  InputPortWidth=3  IndexOptions=Index vector (dialog),Index vector (dialog)  Indices=1,[1 2 3]  OutputSizes=1,1
  Selector2 : Selector  NumberOfDimensions=2  InputPortWidth=3  IndexOptions=Index vector (dialog),Index vector (dialog)  Indices=2,[1 2 3]  OutputSizes=1,1
  Selector3 : Selector  NumberOfDimensions=2  InputPortWidth=3  IndexOptions=Index vector (dialog),Index vector (dialog)  Indices=2,[1 2 3]  OutputSizes=1,1
  Selector4 : Selector  NumberOfDimensions=2  InputPortWidth=3  IndexOptions=Index vector (dialog),Index vector (dialog)  Indices=3,[1 2 3]  OutputSizes=1,1
  Selector5 : Selector  NumberOfDimensions=2  InputPortWidth=3  IndexOptions=Index vector (dialog),Index vector (dialog)  Indices=3,[1 2 3]  OutputSizes=1,1
  Selector6 : Selector  NumberOfDimensions=2  InputPortWidth=3  IndexOptions=Index vector (dialog),Index vector (dialog)  Indices=1,[1 2 3]  OutputSizes=1,1
  Selector8 : Selector  NumberOfDimensions=2  InputPortWidth=3  IndexOptions=Index vector (dialog),Index vector (dialog)  Indices=2,[1 2 3]  OutputSizes=1,1
  Sun position : Subsystem
  Torque arm MB : Subsystem
  Torque arm SP : Subsystem
  Transpose1 : Math  Operator=transpose  SaturateOnIntegerOverflow=on
  Transpose2 : Math  Operator=transpose  SaturateOnIntegerOverflow=on
  Transpose3 : Math  Operator=transpose  SaturateOnIntegerOverflow=on
  M_SRP : Outport
  S_N : Outport  Port=2
  S_B : Outport  Port=3
  wires:
  A_B_N/1 -> Sun position/1(A_B_N)
  Sun position/1(S_B) -> Normalize Vector/1
  Normalize Vector/1 -> [S_B]
  r_SP1/1 -> Torque arm SP/5(r_SP1)
  r_SP2/1 -> Torque arm SP/6(r_SP2)
  MB/1 -> [MB]
  SP/1 -> [SP]
  Sun position/2(S_N) -> [S_N]
  [S_N] -> S_N/1
  N_MB/1 -> Reshape2/1
  S_B dot N_MB/1(MB_illuminated) -> [NMB_true]
  [NMB_true] -> Force MB/2(NMB_true)
  [S_B] -> S_B dot N_MB/2(S_B)
  [MB] -> Areas/1(MB)
  Pressure/1(P) -> [P]
  Areas/1(A_vect) -> [A_vect]
  [P] -> Force MB/1(P)
  [A_vect] -> Force MB/3(A_vect)
  Constant/1 -> Force MB/4(rho_d_MB)
  Constant1/1 -> Force MB/5(rho_s_MB)
  [S_B] -> Reshape/1
  S_B dot N_MB/2(pointer) -> [pointer_MB]
  [pointer_MB] -> Torque arm MB/4(pointer)
  [S_B] -> Torque arm MB/3(S_B)
  [A_vect] -> Torque arm MB/2(A_vect)
  [MB] -> Torque arm MB/1(MB)
  Reshape/1 -> Force MB/6(S_B)
  Cross Product2/1 -> Add/1
  Selector/1 -> Cross Product2/1
  Selector1/1 -> Cross Product2/2
  Selector3/1 -> Cross Product1/2
  Selector2/1 -> Cross Product1/1
  [dist] -> Selector2/1, Selector5/1, Selector/1
  Cross Product1/1 -> Add/2
  Force MB/1(F_MB) -> [F_MB]
  [F_MB] -> Scope1/1, Selector4/1, Selector3/1, Selector1/1
  Cross Product3/1 -> Add/3
  Selector4/1 -> Cross Product3/2
  Selector5/1 -> Cross Product3/1
  Add/1 -> Transpose1/1
  Torque arm MB/1(dist) -> [dist]
  S_B dot N_SP/2(pointer) -> [pointer_SP]
  Areas_SP/1(A_vect) -> [A_vect_SP]
  [SP] -> Areas_SP/1(SP)
  Transpose2/1 -> S_B dot N_SP/2(S_B)
  [S_B] -> Transpose2/1
  S_B dot N_SP/1(SP_illuminated) -> [NSP_true]
  N_SP/1 -> Reshape1/1
  Reshape1/1 -> S_B dot N_SP/1(N_SP)
  Reshape2/1 -> S_B dot N_MB/1(N_MB)
  [P] -> Force SP/1(P)
  [NSP_true] -> Force SP/2(NSP_true)
  [A_vect_SP] -> Force SP/3(A_vect_SP)
  Constant2/1 -> Force SP/4(rho_d_SP)
  Constant3/1 -> Force SP/5(rho_s_SP)
  [S_B] -> Force SP/6(S_B)
  [S_B] -> S_B/1
  [pointer_SP] -> Torque arm SP/4(pointer_SP)
  [SP] -> Torque arm SP/1(SP)
  [A_vect_SP] -> Torque arm SP/2(A_vect_SP)
  [S_B] -> Torque arm SP/3(S_B)
  Torque arm SP/1(distance) -> [dist_SP]
  Force SP/1(F_SP) -> [F_SP]
  Transpose3/1 -> [M_SP]
  Add1/1 -> Transpose3/1
  Cross Product4/1 -> Add1/2
  [dist_SP] -> Selector6/1, Selector8/1
  Selector8/1 -> Cross Product4/1
  [F_SP] -> Cross Product5/2, Cross Product4/2, Scope3/1
  Selector6/1 -> Cross Product5/1
  Cross Product5/1 -> Add1/1
  Transpose1/1 -> [M_MB]
  [M_MB] -> Add2/1
  Add2/1 -> Scope/1, M_SRP/1
  [M_SP] -> Add2/2
